simulink model "SVPWM_7_SEG"  (R2015b)
settings: Solver=ode23  StartTime=0.0  StopTime=0.05  MaxStep=1e-6  RelTol=1e-3
settings Model: Creator=InPower 006  LastModifiedBy=InPower 006

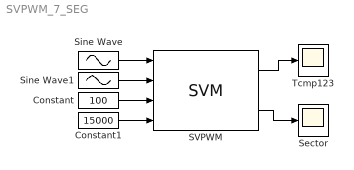
== system SVPWM_7_SEG ==
  Constant : Constant  Value=100
  Constant1 : Constant  Value=15000
  SVPWM : S-Function  InitFcn=try, set_param(gcb,'FunctionName','SVM'), end  FunctionName=SVM  SFunctionModules=SVM_wrapper Svpwm  SFunctionDeploymentMode=off  EnableBusSupport=off  mask(S-Function Builder){}
      mask help: Simulink:masks:SFunctionBuilder_MD
      mask init:
      | val = [[.9  0.75 0.75 1 1 .9 .9 1]',[1 1 0.75 0.75 .9 .9 1 .9]'];try , sys = get_param(gcb,'SfunBuilderFcnName');if isempty(sys), sys = get_param(gcb,'FunctionName'); end,catch, sys = get_param(gcb,'FunctionName'); end
      settings: CopyFcn=set_param(gcbh,'LinkStatus','none')  PreSaveFcn=try, set_param(gcb,'FunctionName','SVM'), end  OpenFcn=sfunctionwizard(gcbh)
      mask Display: plot(val(:,1),val(:,2)),disp(sys), port_label('input',1,'Ualpha'), port_label('input',2,'Ubeta'), port_label('input',3,'Udc'), port_label('input',4,'Tcnt'), port_label('output',1,'Tcmp'), port_label('output',2,'Sec')
  Sector : Scope
  Sine Wave : Sin  Amplitude=50  Frequency=2*pi*50  SampleTime=0
  Sine Wave1 : Sin  Amplitude=50  Frequency=2*pi*50  Phase=-pi/2  SampleTime=0
  Tcmp123 : Scope
  wires:
  Sine Wave/1 -> SVPWM/1
  Sine Wave1/1 -> SVPWM/2
  Constant/1 -> SVPWM/3
  Constant1/1 -> SVPWM/4
  SVPWM/1 -> Tcmp123/1
  SVPWM/2 -> Sector/1
